simulink model "model1"  (R2020b)
settings: Solver=VariableStepAuto  StartTime=0.0  StopTime=10.0  RelTol=1e-3
settings Model: Creator=dkravchenko  LastModifiedBy=dkravchenko

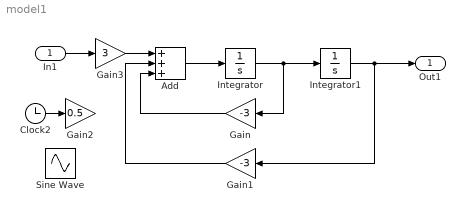
== system model1 ==
  In1 : Inport
  Add : Sum  Inputs=+++
  Clock2 : Clock
  Gain : Gain  Gain=-3
  Gain1 : Gain  Gain=-3
  Gain2 : Gain  Gain=0.5
  Gain3 : Gain  Gain=3
  Integrator : Integrator
  Integrator1 : Integrator  InitialCondition=-1
  Sine Wave : Sin  Frequency=2  SampleTime=0
  Out1 : Outport
  wires:
  Add/1 -> Integrator/1
  Integrator/1 -> Gain/1, Integrator1/1
  Integrator1/1 -> Out1/1, Gain1/1
  Gain1/1 -> Add/2
  Gain/1 -> Add/3
  Clock2/1 -> Gain2/1
  Gain3/1 -> Add/1
  In1/1 -> Gain3/1
